simulink model "ADARTA"  (R2023b)
settings: Solver=FixedStepAuto  StartTime=0  StopTime=9  RelTol=1e-3
values from neighbouring files (symbols this model uses):
  X = [0 -180 -180 -180 180 180 180 180 0]    [Simulaiton_Main.m]    (also in csp_XYZ.m; csp_XYZ_X.m = [-180 -180]; csp_XYZ_circular_motion.m = center(1) + radius * cos(theta); csp_angles.m)
  Y = zeros(1,numel(X_3ars))    [CSPPPPPPPPPPPPpp.m]    (also in Simulaiton_Main.m = zeros(1,9); csp_XYZ.m = zeros(1,9); csp_XYZ_X.m = [0 0]; csp_XYZ_circular_motion.m = center(2) + radius * sin(theta))
  Z = -400*ones(1,numel(X_3ars))    [CSPPPPPPPPPPPPpp.m]    (also in Simulaiton_Main.m = [-300 -300 -400 -300 -300 -300 -400 -300 -300]; csp_XYZ.m = [-300 -300 -400 -300 -300 -300 -400 -300 -300]; csp_XYZ_X.m = [-300 -500]; csp_XYZ_circular_motion.m = center(3) * ones(size(X)))
undefined symbols (not defined in the file or in its folder): smiData
libraries: sm_lib x390, nesl_utility x4
(part 1 of 8)
settings Model: Creator=Dell  LastModifiedBy=Dell

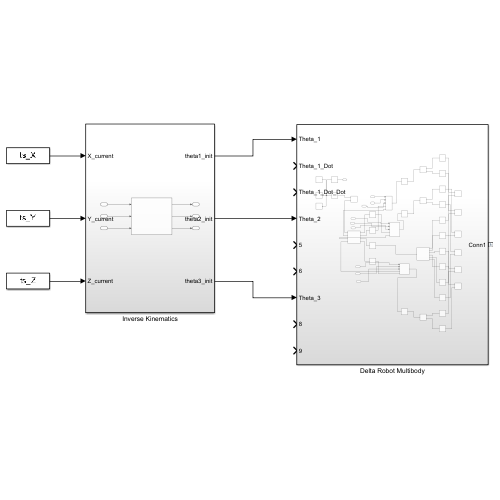
[thumbnail: Simulink's stored preview of the top-level diagram]
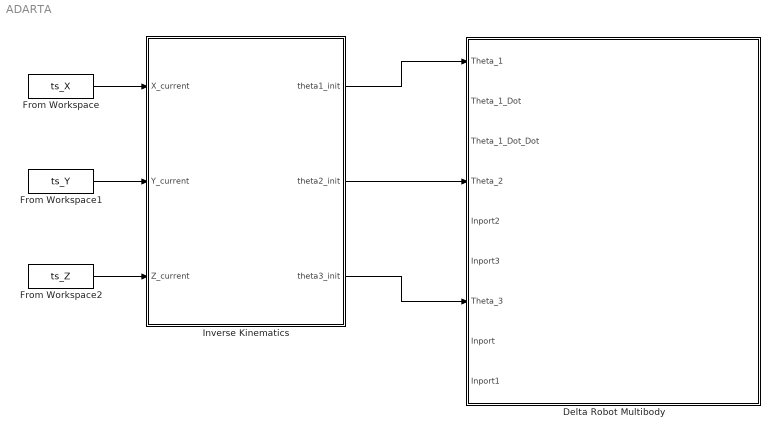
== system ADARTA ==
  Delta Robot Multibody : Subsystem
  From Workspace : FromWorkspace  VariableName=ts_X
  From Workspace1 : FromWorkspace  VariableName=ts_Y
  From Workspace2 : FromWorkspace  VariableName=ts_Z
  Inverse Kinematics : Subsystem
  wires:
  Inverse Kinematics/1(theta1_init) -> Delta Robot Multibody/1(Theta_1)
  Inverse Kinematics/2(theta2_init) -> Delta Robot Multibody/4(Theta_2)
  Inverse Kinematics/3(theta3_init) -> Delta Robot Multibody/7(Theta_3)
  From Workspace/1 -> Inverse Kinematics/1(X_current)
  From Workspace1/1 -> Inverse Kinematics/2(Y_current)
  From Workspace2/1 -> Inverse Kinematics/3(Z_current)
